simulink model "RCAM"  (R2022b)
settings: Solver=VariableStepAuto  StartTime=0.0  StopTime=150  RelTol=1e-3
values from neighbouring files (symbols this model uses):
  u1max = 25*pi/180    (= 0.436332312999)    [initialize_constants_integrator.m]
  u1min = -25*pi/180    (= -0.436332312999)    [initialize_constants_integrator.m]
  u2max = 10*pi/180    (= 0.174532925199)    [initialize_constants_integrator.m]
  u2min = -25*pi/180    (= -0.436332312999)    [initialize_constants_integrator.m]
  u3max = 30*pi/180    (= 0.523598775598)    [initialize_constants_integrator.m]
  u3min = -30*pi/180    (= -0.523598775598)    [initialize_constants_integrator.m]
  u4max = 10*pi/180    (= 0.174532925199)    [initialize_constants_integrator.m]
  u4min = 0    [initialize_constants_integrator.m]
  u5max = 10*pi/180    (= 0.174532925199)    [initialize_constants_integrator.m]
  u5min = 0    [initialize_constants_integrator.m]
  v0 = [0 ... (first row only)    [initialize_constants_integrator.m]
  x0 = [85 ... (first row only)    [initialize_constants_integrator.m]
undefined symbols (not defined in the file or in its folder): RCAM_model
libraries: simulink_extras x5, aerolibfltsims x2, aerolibatmos2 x1, aerolibanim x1
settings Model: Creator=Rahul N  LastModifiedBy=Rahul N

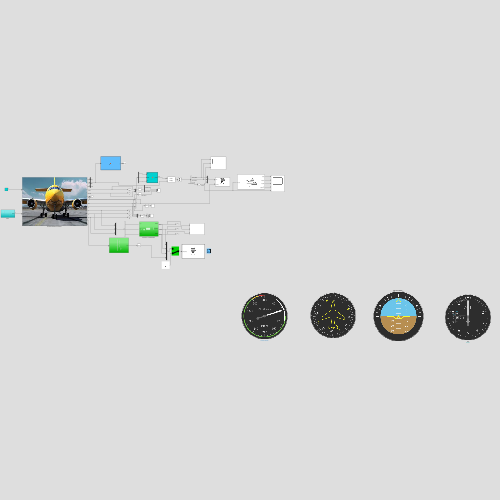
[thumbnail: Simulink's stored preview of the top-level diagram]
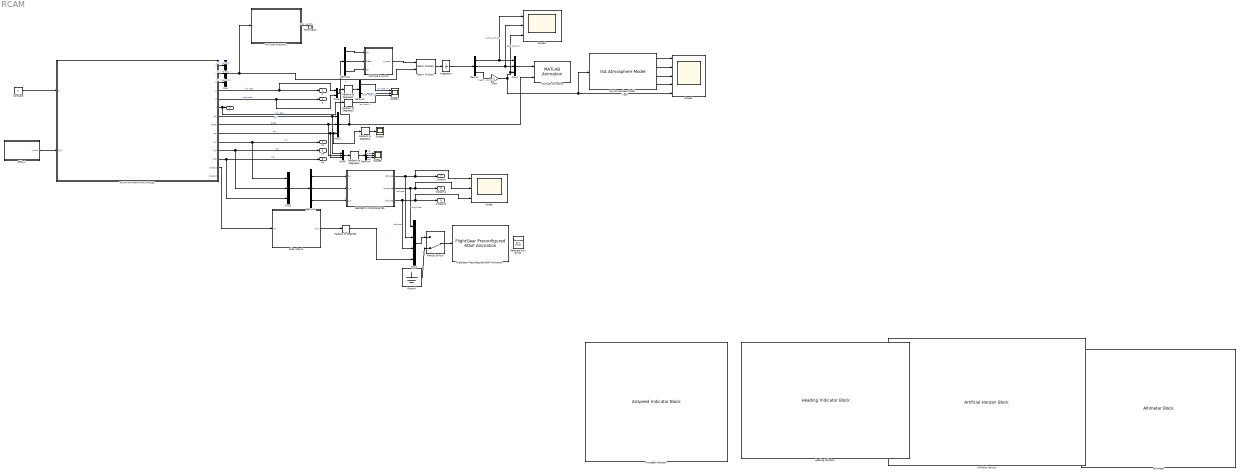
== system RCAM ==
  Airspeed Indicator : AirspeedIndicatorBlock
  Altimeter : AltimeterBlock  LabelPosition=Bottom
  Artificial Horizon : ArtificialHorizonBlock
  Constant : Constant  Value=u
  Demux{,1,3..4} (4 alike) : Demux  Outputs=3
  Demux2 : Demux  Outputs=2
  FlightGear Preconfigured 6DoF Animation : aerolibfltsims/FlightGear Preconfigured 6DoF Animation  xFlightGearVersion=v2019.1  DestinationIpAddress=127.0.0.1  DestinationPort=5502  SampleTime=1/30  packetVersion=24
  "GEODETIC COORDINATES " : Subsystem
  Gain : Gain  Gain=-1
  Generate Run Script : aerolibfltsims/Generate Run Script  Architecture=Win64  dataFlow=Send  GeometryModelName=c172p  AirportId=KSFO  RunwayId=10L  InitialAltitude=2000  InitialHeading=113  OffsetDistance=4.72  OffsetAzimuth=0  InstallScenery=off  DisableShaders=on  OriginAddress=127.0.0.1  DestinationPort=5502  OriginPort=5505  LocalAddress=127.0.0.1  OutputFileName=runfg.bat  FlightGearBaseDirectory=C:\Program Files\FlightGear 2018.1.1
  Ground : Ground
  Heading Indicator : HeadingIndicatorBlock
  ISA Atmosphere Model : aerolibatmos2/ISA Atmosphere Model  custom=on  g=9.80665  gamma=1.4  R=287.0531  L=0.0065  h_trop=11000  h_strat=20000  rho0=1.225  P0=101325  T0=288.15  h0=0
  Integrator : Integrator
  MATLAB Animation : aerolibanim/MATLAB Animation  Tag=Matlab Animation 6 DOF  Vehicles=1  Geometries='pa24-250_orange.ac'  BoundingBoxCoordinates=[-50,50,-50,50,-50,50]  CameraOffset=[-150,-50,0]  CameraViewAngle=3  SampleTime=0.2  FigurePosition=[409,1.858000e+02,6.504000e+02,4.320000e+02]
  MATLAB Function : MATLAB Function  TreatAsAtomicUnit=on
  MATLAB Function1 : MATLAB Function  TreatAsAtomicUnit=on
  Manual Switch : ManualSwitch  CurrentSetting=0
  Matrix Multiply : Product  Multiplication=Matrix(*)
  Mux{,1..3,6} (5 alike) : Mux  Inputs=3
  Mux4 : Mux
  Mux5 : Mux  Inputs=2
  "RCAM MATHEMATICAL MODEL " : Subsystem  Tag=RCAM MATHEMATICAL MODEL  Description=|  mask{Parameter1=|}
      | This subsystem contains the mathematical model of a research civil Aircraft model.
      | It also contains the saturations of controll inputs given to the model, which can be changed by changing saturation values in the initialization script 
      | 
      | It contains blocks and function for determining the north-east-dowm velocity, which is then converted into north east positions with altitude.
      mask Parameter1=|
      | this block contains first 9 state vectors like u v w p q r phi theta psi,
      | with addition of velocity north, velocity east and velcoity down usign direction cosine matrix (DCM)
      |
      | PLEASE LOOK UNDER THE SUBSYSTEM TO MORE ABOUT THE MODEL
      |
      | --PRAJWAL N
      mask prompts: Parameter1 "this block gives the state vectors as output throgh RCAM mathematical model"
      mask Display: image('$imagefile'); % Use "Edit Image" on toolstrip to change.
  Radians to Degrees{,1..4} (5 alike) : simulink_extras/Transformations/Radians to Degrees
  Scope{,2,4..5} (4 alike) : Scope  NumInputPorts=3
  Scope1 : Scope  NumInputPorts=5
  Scope3 : Scope
  Subsystem2 : Subsystem
  Terminator : Terminator
  "delta u " : Subsystem
  p : Outport
  q : Outport  Port=2
  r : Outport  Port=3
  Vn : Outport  Port=4
  Ve : Outport  Port=5
  Vd : Outport  Port=6
  Outport : Outport  Port=7
  Outport1 : Outport  Port=8
  Outport2 : Outport  Port=9
  wires:
  Constant/1 -> "RCAM MATHEMATICAL MODEL "/1(U)
  "delta u "/1(Input1) -> "RCAM MATHEMATICAL MODEL "/2(D_U)
  "RCAM MATHEMATICAL MODEL "/1(u) -> Mux/1  "u ( x velocity )"
  "RCAM MATHEMATICAL MODEL "/2(v) -> Mux/2  "V (y velocity)"
  "RCAM MATHEMATICAL MODEL "/3(w) -> Mux/3  "W ( z velcoity)"
  "RCAM MATHEMATICAL MODEL "/4(p) -> Mux5/1, p/1  "roll rate"
  "RCAM MATHEMATICAL MODEL "/5(q) -> Mux5/2, q/1  "pitch rate"
  "RCAM MATHEMATICAL MODEL "/6(r) -> Radians to Degrees3/1, r/1  "yaw rate"
  "RCAM MATHEMATICAL MODEL "/7(phi) -> Mux6/1, Mux2/1  "phi"
  "RCAM MATHEMATICAL MODEL "/8(theta) -> Mux6/2, Mux2/2  "theta"
  "RCAM MATHEMATICAL MODEL "/9(psi) -> Mux6/3, Radians to Degrees1/1, Mux2/3  "psi"
  "RCAM MATHEMATICAL MODEL "/10(V_N) -> Mux3/1, Vn/1  "V_N"
  "RCAM MATHEMATICAL MODEL "/11(V_E) -> Mux3/2, Ve/1  "V_E"
  "RCAM MATHEMATICAL MODEL "/12(V_D) -> Mux3/3, Vd/1  "V_D"
  MATLAB Function/1(r_matrix) -> Matrix Multiply/1
  Matrix Multiply/1 -> Integrator/1
  Integrator/1 -> Demux/1
  Demux/1 -> Scope2/1, Mux1/1  "north position"
  Demux/2 -> Scope2/2, Mux1/2  "east position"
  Demux/3 -> Gain/1  "hiegth  position"
  Mux2/1 -> Demux3/1, MATLAB Animation/2
  Mux1/1 -> MATLAB Animation/1
  Gain/1 -> Scope2/3, Mux1/3, Scope1/5, ISA Atmosphere Model/1  "hiegth"
  Mux3/1 -> Demux1/1
  Demux1/1 -> "GEODETIC COORDINATES "/1(V_n)
  Demux1/2 -> "GEODETIC COORDINATES "/2(V_e)
  Demux1/3 -> "GEODETIC COORDINATES "/3(V_d)
  "GEODETIC COORDINATES "/1(latitude) -> Mux4/2, Scope/1, Outport/1  "latitude"
  "GEODETIC COORDINATES "/2(longitude) -> Scope/2, Outport1/1, Mux4/1  "longitude"
  "GEODETIC COORDINATES "/3(altitude) -> Scope/3, Outport2/1, Mux4/3  "altitude"
  "RCAM MATHEMATICAL MODEL "/13(Output) -> Subsystem2/1(In1)
  Subsystem2/1(phi1) -> Radians to Degrees/1
  Mux4/1 -> Manual Switch/1
  Ground/1 -> Manual Switch/2
  Manual Switch/1 -> FlightGear Preconfigured 6DoF Animation/1
  Radians to Degrees/1 -> Mux4/4
  Mux/1 -> MATLAB Function1/1(s), Matrix Multiply/2  "s"
  ISA Atmosphere Model/1 -> Scope1/1
  ISA Atmosphere Model/2 -> Scope1/2
  ISA Atmosphere Model/3 -> Scope1/3
  ISA Atmosphere Model/4 -> Scope1/4
  MATLAB Function1/1(y) -> Terminator/1  "total velocity"
  Radians to Degrees1/1 -> Scope3/1
  Mux5/1 -> Radians to Degrees2/1
  Demux2/1 -> Scope4/1  "roll rate (p)"
  Demux2/2 -> Scope4/2  "pitch rate (q)"
  Radians to Degrees2/1 -> Demux2/1
  Demux3/1 -> MATLAB Function/1(phi)
  Demux3/2 -> MATLAB Function/2(theta)
  Demux3/3 -> MATLAB Function/3(psi)
  Radians to Degrees3/1 -> Scope4/3  "yaw rate (r)"
  Mux6/1 -> Radians to Degrees4/1
  Radians to Degrees4/1 -> Demux4/1
  Demux4/1 -> Scope5/1  "phi"
  Demux4/2 -> Scope5/2  "theta"
  Demux4/3 -> Scope5/3  "psi"

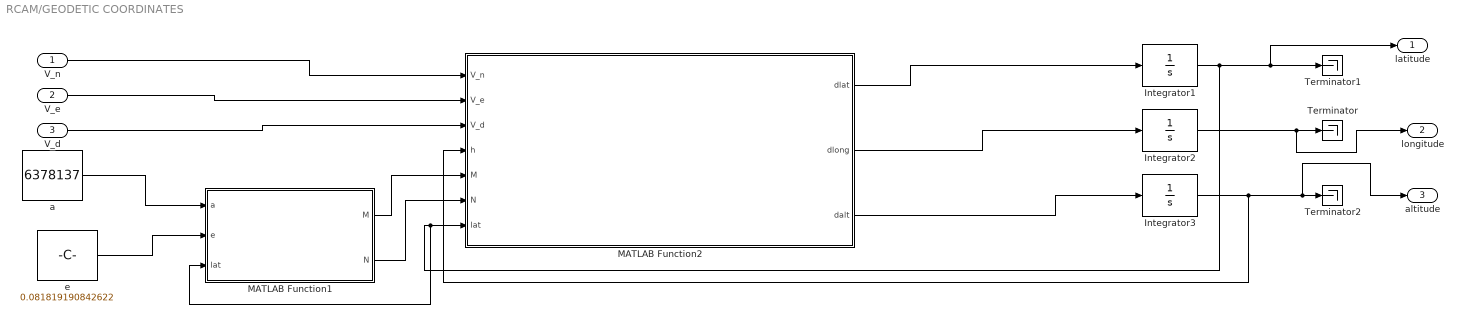
== system RCAM/GEODETIC COORDINATES  ==
  V_n : Inport
  V_e : Inport  Port=2
  V_d : Inport  Port=3
  Integrator1 : Integrator
  Integrator2 : Integrator
  Integrator3 : Integrator
  MATLAB Function1 : MATLAB Function  TreatAsAtomicUnit=on
  MATLAB Function2 : MATLAB Function  TreatAsAtomicUnit=on
  Terminator : Terminator
  Terminator1 : Terminator
  Terminator2 : Terminator
  a : Constant  Value=6378137
  e : Constant  Value=0.081819190842622
  latitude : Outport
  longitude : Outport  Port=2
  altitude : Outport  Port=3
  wires:
  MATLAB Function2/3(dalt) -> Integrator3/1
  Integrator3/1 -> MATLAB Function2/4(h), altitude/1, Terminator2/1
  a/1 -> MATLAB Function1/1(a)
  Integrator2/1 -> longitude/1, Terminator/1
  MATLAB Function2/2(dlong) -> Integrator2/1
  V_n/1 -> MATLAB Function2/1(V_n)
  Integrator1/1 -> latitude/1, Terminator1/1, MATLAB Function1/3(lat), MATLAB Function2/7(lat)
  e/1 -> MATLAB Function1/2(e)
  MATLAB Function1/1(M) -> MATLAB Function2/5(M)
  MATLAB Function1/2(N) -> MATLAB Function2/6(N)
  MATLAB Function2/1(dlat) -> Integrator1/1
  V_e/1 -> MATLAB Function2/2(V_e)
  V_d/1 -> MATLAB Function2/3(V_d)

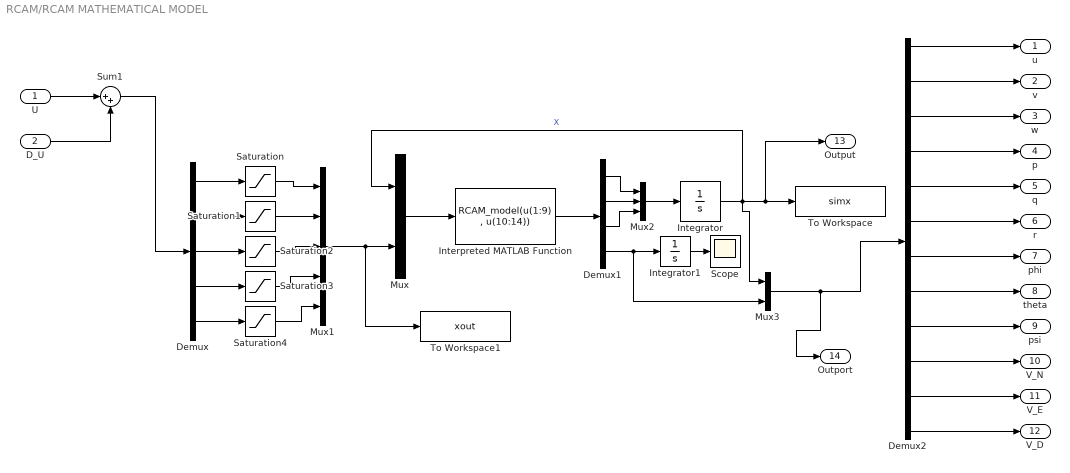
== system RCAM/RCAM MATHEMATICAL MODEL  ==
  U : Inport
  D_U : Inport  Port=2
  Demux : Demux  Outputs=5
  Demux1 : Demux
  Demux2 : Demux  Outputs=12
  Integrator : Integrator  InitialCondition=x0
  Integrator1 : Integrator  InitialCondition=v0
  Interpreted MATLAB Function : MATLABFcn  MATLABFcn=RCAM_model(u(1:9) , u(10:14))
  Mux : Mux  Inputs=2
  Mux1 : Mux  Inputs=5
  Mux2 : Mux  Inputs=3
  Mux3 : Mux  Inputs=2
  Saturation : Saturate  UpperLimit=u1max  LowerLimit=u1min
  Saturation1 : Saturate  UpperLimit=u2max  LowerLimit=u2min
  Saturation2 : Saturate  UpperLimit=u3max  LowerLimit=u3min
  Saturation3 : Saturate  UpperLimit=u4max  LowerLimit=u4min
  Saturation4 : Saturate  UpperLimit=u5max  LowerLimit=u5min
  Scope : Scope
  Sum1 : Sum  Inputs=|++
  To Workspace : ToWorkspace  VariableName=simx  SaveFormat=Timeseries  SampleTime=-1
  To Workspace1 : ToWorkspace  VariableName=xout  SaveFormat=Timeseries  SampleTime=-1
  u : Outport
  v : Outport  Port=2
  w : Outport  Port=3
  p : Outport  Port=4
  q : Outport  Port=5
  r : Outport  Port=6
  phi : Outport  Port=7
  theta : Outport  Port=8
  psi : Outport  Port=9
  V_N : Outport  Port=10
  V_E : Outport  Port=11
  V_D : Outport  Port=12
  Output : Outport  Port=13
  Outport : Outport  Port=14
  wires:
  Demux/5 -> Saturation4/1
  Mux/1 -> Interpreted MATLAB Function/1
  Integrator/1 -> Output/1, To Workspace/1, Mux/1, Mux3/1  "X"
  U/1 -> Sum1/1
  Mux1/1 -> Mux/2, To Workspace1/1
  Integrator1/1 -> Scope/1
  Mux2/1 -> Integrator/1
  Demux1/2 -> Mux2/2
  Sum1/1 -> Demux/1
  Demux/2 -> Saturation1/1
  Demux/1 -> Saturation/1
  Demux/3 -> Saturation2/1
  Demux2/10 -> V_N/1
  Demux2/4 -> p/1
  Demux/4 -> Saturation3/1
  Saturation2/1 -> Mux1/3
  Saturation4/1 -> Mux1/5
  Saturation1/1 -> Mux1/2
  Saturation/1 -> Mux1/1
  Demux2/8 -> theta/1
  Interpreted MATLAB Function/1 -> Demux1/1
  Demux2/6 -> r/1
  Saturation3/1 -> Mux1/4
  Demux1/3 -> Mux2/3
  Demux1/4 -> Mux3/2, Integrator1/1
  Demux1/1 -> Mux2/1
  Demux2/3 -> w/1
  Demux2/2 -> v/1
  Demux2/9 -> psi/1
  Demux2/7 -> phi/1
  Demux2/12 -> V_D/1
  Demux2/11 -> V_E/1
  Demux2/5 -> q/1
  D_U/1 -> Sum1/2
  Demux2/1 -> u/1
  Mux3/1 -> Outport/1, Demux2/1

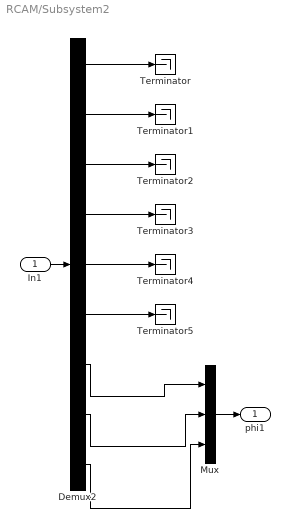
== system RCAM/Subsystem2 ==
  In1 : Inport
  Demux2 : Demux  Outputs=9
  Mux : Mux  Inputs=3
  Terminator{,1..5} (6 alike) : Terminator
  phi1 : Outport
  wires:
  Demux2/4 -> Terminator3/1
  Demux2/2 -> Terminator1/1
  Demux2/1 -> Terminator/1
  In1/1 -> Demux2/1
  Demux2/7 -> Mux/1
  Demux2/5 -> Terminator4/1
  Demux2/3 -> Terminator2/1
  Demux2/6 -> Terminator5/1
  Demux2/8 -> Mux/2
  Demux2/9 -> Mux/3
  Mux/1 -> phi1/1

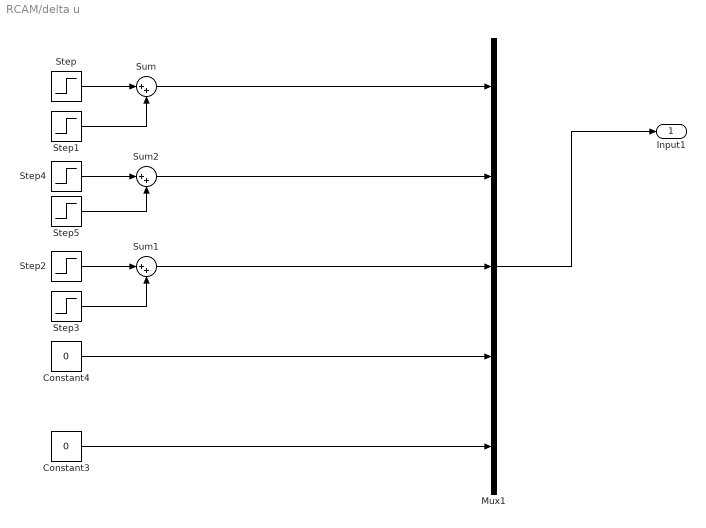
== system RCAM/delta u  ==
  Constant3 : Constant  Value=0
  Constant4 : Constant  Value=0
  Mux1 : Mux  Inputs=5
  Step : Step  Time=10  After=0  SampleTime=0
  Step1 : Step  Time=15  After=0  SampleTime=0
  Step2 : Step  Time=12  After=-6*pi/180  SampleTime=0
  Step3 : Step  Time=17  After=6*pi/180  SampleTime=0
  Step4 : Step  Time=20  After=10*pi/180  SampleTime=0
  Step5 : Step  Time=20 + 5  After=-10*pi/180  SampleTime=0
  Sum : Sum  Inputs=|++
  Sum1 : Sum  Inputs=|++
  Sum2 : Sum  Inputs=|++
  Input1 : Outport
  wires:
  Constant3/1 -> Mux1/5
  Sum/1 -> Mux1/1
  Step1/1 -> Sum/2
  Step/1 -> Sum/1
  Constant4/1 -> Mux1/4
  Mux1/1 -> Input1/1
  Step2/1 -> Sum1/1
  Step3/1 -> Sum1/2
  Sum1/1 -> Mux1/3
  Step4/1 -> Sum2/1
  Step5/1 -> Sum2/2
  Sum2/1 -> Mux1/2

== matlab function RCAM/GEODETIC COORDINATES /MATLAB Function1 ==
  data: a input; M output; e input; lat input; N output
function [M,N] = Meridian_and_primevertical(a,e,lat)

M = (a*(1-e^2))/(1-e^2 * (sin(lat)^2))^(3/2);

N = (a)/(1-e^2 * sin(lat)^2)^(1/2);

end

== matlab function RCAM/MATLAB Function ==
  data: phi input; r_matrix output; theta input; psi input
function r_matrix = R_matrix(phi,theta,psi)

C1v = [cos(psi) -sin(psi) 0 ;
    sin(psi) cos(psi) 0 ;
    0 0 1];

C21 = [ cos(theta) 0 -sin(theta) ;
    0 1 0 ;
    sin(theta) 0 cos(theta)];

Cb2 = [ 1 0 0 ;
    0 cos(phi) sin(phi);
    0 -sin(phi) cos(phi)];

Cbv = C1v*C21*Cb2;

Cvb = Cbv';

r_matrix = Cvb;


end

== matlab function RCAM/GEODETIC COORDINATES /MATLAB Function2 ==
  data: V_n input; dlat output; V_e input; V_d input; h input; M input; N input; lat input; dlong output; dalt output
function [dlat,dlong,dalt] = geodetic_coordinates(V_n,V_e,V_d,h,M ,N ,lat)

dlat = (V_n/(M + h));

dlong = (V_e/(N + h ) * cos(lat));

dalt = -V_d;


end

== matlab function RCAM/MATLAB Function1 ==
  data: s input; y output
function y = total_velocity(s) 

V = sqrt(s(1)^2 + s(2)^2 + s(3)^2);



y = V;

end
